simulink model "libdumbac"  (R2020a)
settings: Solver=FixedStepDiscrete  StartTime=0.0  StopTime=86400  FixedStep=10  RelTol=1e-3
values from neighbouring files (symbols this model uses):
  conE = [ ... (first row only)    [acMdl.m]
  t0filt = Hd.Numerator ./ sum(Hd.Numerator)    [acMdl.m]
libraries: mpclib x1, cstblocks x1
settings Model: Creator=iorioikawa  LastModifiedBy=iorioikawa
settings DataIOCC: SaveOutput=off  SaveTime=off
settings OptimizationCC: DefaultParameterBehavior=Inlined  UseDivisionForNetSlopeComputation=on  GainParamInheritBuiltInType=on  UseFloatMulNetSlope=on  InlineInvariantSignals=on  PassReuseOutputArgsAs=Individual arguments  ZeroExternalMemoryAtStartup=off  ZeroInternalMemoryAtStartup=off  NoFixptDivByZeroProtection=on  EfficientFloat2IntCast=on  LifeSpan=365  OptimizeBlockOrder=speed  DifferentSizesBufferReuse=on  EfficientTunableParamExpr=on
settings DebuggingCC: ParameterTunabilityLossMsg=error
settings HardwareCC: ProdBitPerPointer=32  ProdBitPerSizeT=32  ProdBitPerPtrDiffT=32  ProdLargestAtomicInteger=Long  ProdWordSize=32  ProdLongLongMode=on  ProdHWDeviceType=ARM Compatible->ARM 7
settings SFSimCC: MATLABDynamicMemAlloc=off
settings RTWCC: SystemTargetFile=ert.tlc  GenCodeOnly=on  TemplateMakefile=ert_default_tmf  TargetLang=C++
settings CodeAppCC: ForceParamTrailComments=on  IgnoreCustomStorageClasses=off  OperatorAnnotations=on  SimulinkDataObjDesc=on  SFDataObjDesc=on  CustomSymbolStrGlobalVar=rt$N$M  CustomSymbolStrType=$N$M  CustomSymbolStrFcn=$N$M$F  CustomSymbolStrMacro=$N$M  InsertBlockDesc=on
settings ERTTargetCC: TargetLangStandard=C++03 (ISO)  GenerateSampleERTMain=on  IncludeMdlTerminateFcn=off  CombineSignalStateStructs=on  SupportAbsoluteTime=off  MultiInstanceERTCode=on  CodeInterfacePackaging=C++ class  SupportComplex=off  SupportNonInlinedSFcns=on  InlinedParameterPlacement=NonHierarchical  RootIOFormat=Structure reference  RTWCAPISignals=on  ERTCustomFileTemplate=example_file_process.tlc  ERTFilePackagingFormat=CompactWithDataFile  IndentStyle=Allman  IndentSize=4

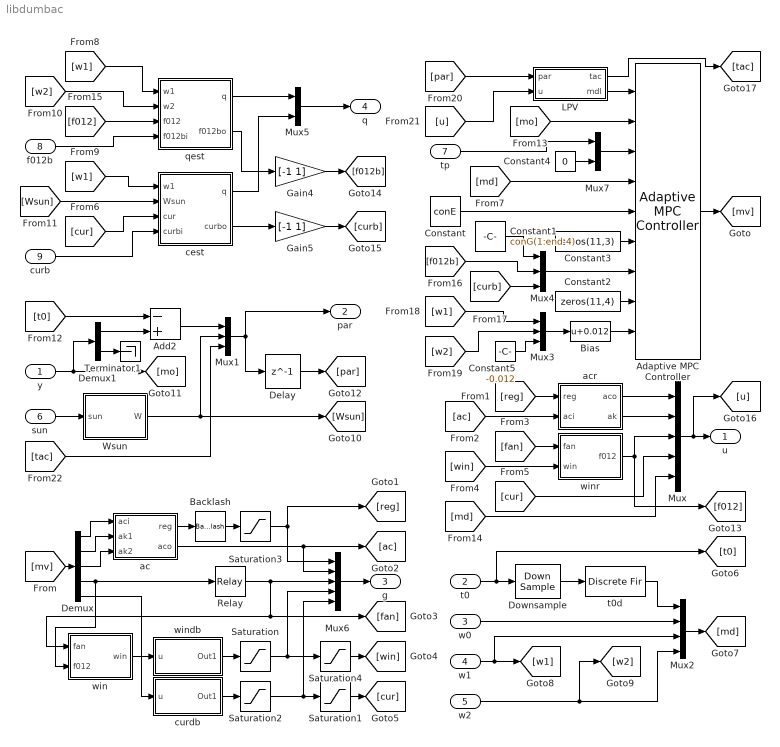
== system libdumbac ==
  y : Inport  OutDataTypeStr=double  PortDimensions=2  SampleTime=10
  t0 : Inport  Port=2  OutDataTypeStr=double  PortDimensions=1  SampleTime=10
  w0 : Inport  Port=3  OutDataTypeStr=double  PortDimensions=1  SampleTime=10
  w1 : Inport  Port=4  OutDataTypeStr=double  PortDimensions=1  SampleTime=10
  w2 : Inport  Port=5  OutDataTypeStr=double  PortDimensions=1  SampleTime=10
  sun : Inport  Port=6  OutDataTypeStr=double  PortDimensions=3  SampleTime=10
  tp : Inport  Port=7  OutDataTypeStr=double  PortDimensions=2  SampleTime=10
  f012b : Inport  Port=8  OutDataTypeStr=double  PortDimensions=2  SampleTime=10
  curb : Inport  Port=9  OutDataTypeStr=double  PortDimensions=2  SampleTime=10
  Adaptive MPC Controller : mpclib/Adaptive MPC Controller  SCDEnableBlockLinearizationSpecification=on  mpcobj=Gdsam  enable_value=0  updateMPCinCallerWorkspace=on  md_inport=on  mv_inport=off  uref_inport=off  return_cost=off  return_mvseq=off  return_qpstatus=off  return_xseq=off  return_state=off  return_ovseq=off  state_inport=off  isltv_plant=off  umin_inport=off  umax_inport=off  ymin_inport=off  ymax_inport=off  cc_inport=on  ywt_inport=on  uwt_inport=off  duwt_inport=off  rhoeps_inport=off  pm_inport=off  MaximumP=10  HorizonChoice=FixedHorizon  BlockDataType=double  SampleTimeInherited=off  switch_inport=off
  Add2 : Sum  Inputs=-+
  Backlash : Backlash  BacklashWidth=0.005
  Bias : Bias  Bias=0.012
  Constant : Constant  Value=conE
  Constant1 : Constant  Value=conG(1:end-4)
  Constant2 : Constant  Value=zeros(11,4)
  Constant3 : Constant  Value=zeros(11,3)
  Constant4 : Constant  Value=0
  Constant5 : Constant  Value=-0.012
  Delay : Delay  DelayLength=1  InitialCondition=0
  Demux : Demux  Outputs=5
  Demux1 : Demux  Outputs=2
  Downsample : DownSample  N=60
  Gain4 : Gain  Gain=[-1 1]
  Gain5 : Gain  Gain=[-1 1]
  LPV : Subsystem
  Mux : Mux  Inputs=5
  Mux1 : Mux  Inputs=3
  Mux2 : Mux
  Mux3 : Mux  Inputs=3
  Mux4 : Mux  Inputs=3
  Mux5 : Mux  Inputs=2
  Mux6 : Mux  Inputs=5
  Mux7 : Mux  Inputs=2
  Relay : Relay  OnSwitchValue=0.2  OffSwitchValue=0.1
  Saturation : Saturate  UpperLimit=1  LowerLimit=-0.1
  Saturation1 : Saturate  UpperLimit=1  LowerLimit=0
  Saturation2 : Saturate  UpperLimit=1  LowerLimit=-0.1
  Saturation3 : Saturate  UpperLimit=2  LowerLimit=0
  Saturation4 : Saturate  UpperLimit=1  LowerLimit=0
  Terminator1 : Terminator
  Wsun : MATLAB Function  TreatAsAtomicUnit=on
  ac : Subsystem
  acr : MATLAB Function  TreatAsAtomicUnit=on
  cest : Subsystem
  curdb : Subsystem
  qest : Subsystem
  t0d : DiscreteFir  Coefficients=t0filt
  win : MATLAB Function  TreatAsAtomicUnit=on
  windb : Subsystem
  winr : MATLAB Function  TreatAsAtomicUnit=on
  u : Outport  OutDataTypeStr=double  PortDimensions=9  SampleTime=10
  par : Outport  Port=2  OutDataTypeStr=double  PortDimensions=3  SampleTime=10
  g : Outport  Port=3  OutDataTypeStr=double  PortDimensions=8  SampleTime=10
  q : Outport  Port=4  OutDataTypeStr=double  PortDimensions=2  SampleTime=10
  wires:
  Mux1/1 -> par/1, Delay/1
  w1/1 -> [w1], Mux2/3
  w2/1 -> Mux2/4, [w2]
  Mux3/1 -> Bias/1
  Add2/1 -> Mux1/1
  t0d/1 -> Mux2/1
  Bias/1 -> Adaptive MPC Controller/9
  y/1 -> Demux1/1, [mo]
  w0/1 -> Mux2/2
  t0/1 -> [t0], Downsample/1
  Demux1/1 -> Add2/2
  sun/1 -> Wsun/1(sun)
  Demux1/2 -> Terminator1/1
  Mux/1 -> [u], u/1
  Delay/1 -> [par]
  acr/1(aco) -> Mux/1
  acr/2(ak) -> Mux/2
  Demux/5 -> curdb/1(u)
  Demux/4 -> win/2(f012), Relay/1
  Relay/1 -> Mux6/3, [fan], win/1(fan)
  win/1(win) -> windb/1(u)
  curdb/1(Out1) -> Saturation2/1
  windb/1(Out1) -> Saturation/1
  Saturation/1 -> Saturation4/1, Mux6/4
  ac/2(aco) -> [ac], Mux6/2
  Saturation2/1 -> Mux6/5, Saturation1/1
  Backlash/1 -> Saturation3/1
  winr/1(f012) -> Mux/3, [f012]
  Mux6/1 -> g/1
  Saturation3/1 -> [reg], Mux6/1
  Demux/1 -> ac/1(aci)
  Demux/2 -> ac/2(ak1)
  ac/1(reg) -> Backlash/1
  Saturation1/1 -> [cur]
  Downsample/1 -> t0d/1
  f012b/1 -> qest/4(f012bi)
  Constant/1 -> Adaptive MPC Controller/5
  Constant2/1 -> Adaptive MPC Controller/8
  Constant3/1 -> Adaptive MPC Controller/6
  Mux4/1 -> Adaptive MPC Controller/7
  Constant1/1 -> Mux4/1
  qest/2(f012bo) -> Gain4/1
  cest/2(curbo) -> Gain5/1
  Mux5/1 -> q/1
  qest/1(q) -> Mux5/1
  cest/1(q) -> Mux5/2
  curb/1 -> cest/4(curbi)
  Adaptive MPC Controller/1 -> [mv]
  [mv] -> Demux/1
  [reg] -> acr/1(reg)
  [ac] -> acr/2(aci)
  [fan] -> winr/1(fan)
  Saturation4/1 -> [win]
  [win] -> winr/2(win)
  [cur] -> cest/3(cur)
  [cur] -> Mux/4
  Mux2/1 -> [md]
  [md] -> Adaptive MPC Controller/4
  [w1] -> qest/1(w1)
  [w1] -> cest/1(w1)
  [w2] -> qest/2(w2)
  Wsun/1(W) -> [Wsun], Mux1/2
  [Wsun] -> cest/2(Wsun)
  [t0] -> Add2/1
  [mo] -> Adaptive MPC Controller/2
  [md] -> Mux/5
  [f012] -> qest/3(f012)
  Gain4/1 -> [f012b]
  [f012b] -> Mux4/2
  Gain5/1 -> [curb]
  [curb] -> Mux4/3
  [w1] -> Mux3/1
  [w2] -> Mux3/2
  [par] -> LPV/1(par)
  LPV/2(mdl) -> Adaptive MPC Controller/1
  Demux/3 -> ac/3(ak2)
  [u] -> LPV/2(u)
  LPV/1(tac) -> [tac]
  [tac] -> Mux1/3
  Mux7/1 -> Adaptive MPC Controller/3
  tp/1 -> Mux7/1
  Constant4/1 -> Mux7/2
  Constant5/1 -> Mux3/3

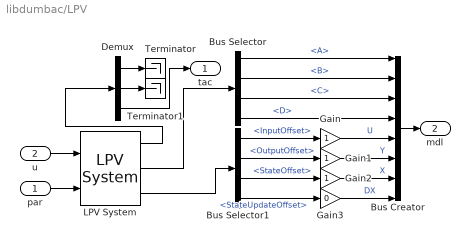
== system libdumbac/LPV ==
  par : Inport
  u : Inport  Port=2
  Bus Creator : BusCreator  Inputs=8
  Bus Selector : BusSelector  OutputSignals=A,B,C,D
  Bus Selector1 : BusSelector  OutputSignals=InputOffset,OutputOffset,StateOffset,StateUpdateOffset
  Demux : Demux  Outputs=3
  Gain : Gain
  Gain1 : Gain
  Gain2 : Gain
  Gain3 : Gain  Gain=0
  LPV System : cstblocks/Linear Parameter Varying/LPV System  sys=Gds  x0=0  uOffset=0  yOffset=0  xOffset=0  opEquilOption=on  dxOffset=0  sysFixedOption=Use the first model in state-space array  sysFixed=[]  AFixed=true  BFixed=false  CFixed=true  DFixed=true  uDelayFixed=true  yDelayFixed=true  iDelayFixed=true  IMethod=Linear  EMethod=Clip  IndexSearch=Linear search  IndexBegin=on  OutputX=off  OutputXdot=off  OutputLTI=on  OutputOP=on  DataType=double  SimMode=Interpreted execution  InitBufferSize=1024  FixedBuffer=off
      settings: SourceProductBaseCode=CT
  Terminator : Terminator
  Terminator1 : Terminator
  tac : Outport
  mdl : Outport  Port=2
  wires:
  u/1 -> LPV System/1
  LPV System/1 -> Demux/1
  Bus Selector/1 -> Bus Creator/1  "<A>"
  Bus Selector1/3 -> Gain2/1  "<StateOffset>"
  Bus Selector/2 -> Bus Creator/2  "<B>"
  Gain2/1 -> Bus Creator/7  "X"
  LPV System/3 -> Bus Selector1/1
  Gain1/1 -> Bus Creator/6  "Y"
  Bus Selector1/1 -> Gain/1  "<InputOffset>"
  Bus Selector/4 -> Bus Creator/4  "<D>"
  par/1 -> LPV System/2
  Gain/1 -> Bus Creator/5  "U"
  LPV System/2 -> Bus Selector/1
  Gain3/1 -> Bus Creator/8  "DX"
  Bus Selector1/2 -> Gain1/1  "<OutputOffset>"
  Bus Selector/3 -> Bus Creator/3  "<C>"
  Bus Creator/1 -> mdl/1
  Bus Selector1/4 -> Gain3/1  "<StateUpdateOffset>"
  Demux/1 -> Terminator/1
  Demux/2 -> Terminator1/1
  Demux/3 -> tac/1

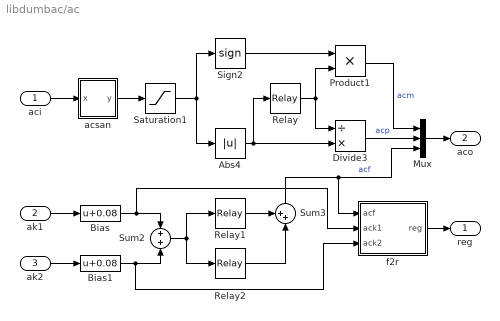
== system libdumbac/ac ==
  aci : Inport
  ak1 : Inport  Port=2
  ak2 : Inport  Port=3
  Abs4 : Abs
  Bias : Bias  Bias=0.08
  Bias1 : Bias  Bias=0.08
  Divide3 : Product  Inputs=/*
  Mux : Mux  Inputs=3
  Product1 : Product
  Relay : Relay  OnSwitchValue=1  OffSwitchValue=0.9  OnOutputValue=2  OffOutputValue=1
  Relay1 : Relay  OnSwitchValue=0.8  OffSwitchValue=0.7
  Relay2 : Relay  OnSwitchValue=0.65  OffSwitchValue=0.55
  Saturation1 : Saturate  UpperLimit=2  LowerLimit=-2
  Sign2 : Signum
  Sum2 : Sum  Inputs=+|+
  Sum3 : Sum  Inputs=++|
  acsan : Subsystem
  f2r : MATLAB Function  TreatAsAtomicUnit=on
  reg : Outport
  aco : Outport  Port=2
  wires:
  f2r/1(reg) -> reg/1
  acsan/1(y) -> Saturation1/1
  aci/1 -> acsan/1(x)
  Saturation1/1 -> Abs4/1, Sign2/1
  Abs4/1 -> Relay/1, Divide3/2
  Divide3/1 -> Mux/2  "acp"
  Product1/1 -> Mux/1  "acm"
  Mux/1 -> aco/1
  Relay/1 -> Divide3/1, Product1/2
  Sign2/1 -> Product1/1
  ak1/1 -> Bias/1
  ak2/1 -> Bias1/1
  Sum2/1 -> Relay1/1, Relay2/1
  Relay1/1 -> Sum3/1
  Relay2/1 -> Sum3/2
  Sum3/1 -> f2r/1(acf), Mux/3  "acf"
  Bias/1 -> f2r/2(ack1), Sum2/1
  Bias1/1 -> f2r/3(ack2), Sum2/2

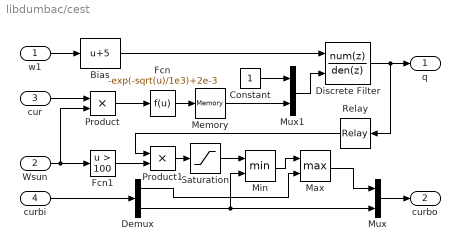
== system libdumbac/cest ==
  w1 : Inport
  Wsun : Inport  Port=2
  cur : Inport  Port=3
  curbi : Inport  Port=4
  Bias : Bias  Bias=5
  Constant : Constant
  Demux : Demux  Outputs=2
  Discrete Filter : DiscreteFilter  Numerator=9e-4  DenominatorSource=Input port  Denominator=[1 -1]  a0EqualsOne=on
      settings: InputPortMap=u0,p3
  Fcn : Fcn  Expr=-exp(-sqrt(u)/1e3)+2e-3
  Fcn1 : Fcn  Expr=u > 100
  Max : MinMax  Function=max  Inputs=2
  Memory : Memory
  Min : MinMax  Inputs=2
  Mux : Mux  Inputs=2
  Mux1 : Mux  Inputs=2
  Product : Product
  Product1 : Product
  Relay : Relay  OnSwitchValue=2  OffSwitchValue=0.2  OnOutputValue=0.15
  Saturation : Saturate  UpperLimit=1  LowerLimit=0
  q : Outport
  curbo : Outport  Port=2
  wires:
  Discrete Filter/1 -> q/1, Relay/1
  w1/1 -> Bias/1
  curbi/1 -> Demux/1
  Mux/1 -> curbo/1
  Demux/2 -> Mux/2, Min/2
  Demux/1 -> Max/2
  Max/1 -> Mux/1
  Min/1 -> Max/1
  Fcn/1 -> Memory/1
  Mux1/1 -> Discrete Filter/2
  Constant/1 -> Mux1/1
  Memory/1 -> Mux1/2
  Bias/1 -> Discrete Filter/1
  Product/1 -> Fcn/1
  Wsun/1 -> Product/2, Fcn1/1
  Relay/1 -> Product1/1
  Fcn1/1 -> Product1/2
  cur/1 -> Product/1
  Product1/1 -> Saturation/1
  Saturation/1 -> Min/1

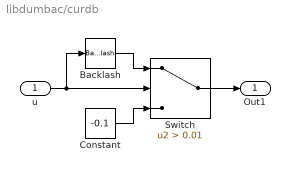
== system libdumbac/curdb ==
  u : Inport
  Backlash : Backlash  BacklashWidth=0.05
  Constant : Constant  Value=-0.1
  Switch : Switch  Criteria=u2 > Threshold  Threshold=0.01
  Out1 : Outport
  wires:
  Constant/1 -> Switch/3
  Switch/1 -> Out1/1
  Backlash/1 -> Switch/1
  u/1 -> Backlash/1, Switch/2

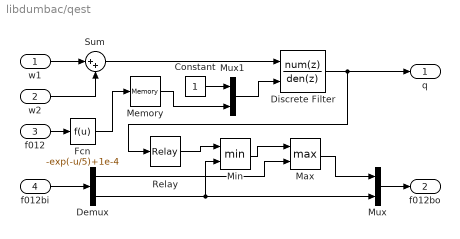
== system libdumbac/qest ==
  w1 : Inport
  w2 : Inport  Port=2
  f012 : Inport  Port=3
  f012bi : Inport  Port=4
  Constant : Constant
  Demux : Demux  Outputs=2
  Discrete Filter : DiscreteFilter  Numerator=1e-3  DenominatorSource=Input port  Denominator=[1 -1]  a0EqualsOne=on
      settings: InputPortMap=u0,p3
  Fcn : Fcn  Expr=-exp(-u/5)+1e-4
  Max : MinMax  Function=max  Inputs=2
  Memory : Memory
  Min : MinMax  Inputs=2
  Mux : Mux  Inputs=2
  Mux1 : Mux  Inputs=2
  Relay : Relay  OnSwitchValue=2  OffSwitchValue=0.2
  Sum : Sum  Inputs=|++
  q : Outport
  f012bo : Outport  Port=2
  wires:
  Discrete Filter/1 -> q/1, Relay/1
  w1/1 -> Sum/1
  w2/1 -> Sum/2
  f012/1 -> Fcn/1
  Relay/1 -> Min/1
  f012bi/1 -> Demux/1
  Mux/1 -> f012bo/1
  Demux/2 -> Mux/2, Min/2
  Demux/1 -> Max/2
  Max/1 -> Mux/1
  Min/1 -> Max/1
  Fcn/1 -> Memory/1
  Mux1/1 -> Discrete Filter/2
  Constant/1 -> Mux1/1
  Memory/1 -> Mux1/2
  Sum/1 -> Discrete Filter/1

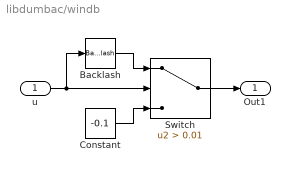
== system libdumbac/windb ==
  u : Inport
  Backlash : Backlash  BacklashWidth=0.05
  Constant : Constant  Value=-0.1
  Switch : Switch  Criteria=u2 > Threshold  Threshold=0.01
  Out1 : Outport
  wires:
  Constant/1 -> Switch/3
  Switch/1 -> Out1/1
  Backlash/1 -> Switch/1
  u/1 -> Backlash/1, Switch/2

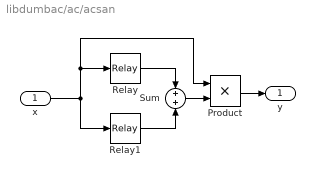
== system libdumbac/ac/acsan ==
  x : Inport
  Product : Product
  Relay : Relay  OnSwitchValue=0.4  OffSwitchValue=0.2
  Relay1 : Relay  OnSwitchValue=-0.2  OffSwitchValue=-0.4  OnOutputValue=0  OffOutputValue=1
  Sum : Sum  Inputs=+|+
  y : Outport
  wires:
  Product/1 -> y/1
  Sum/1 -> Product/2
  Relay1/1 -> Sum/2
  Relay/1 -> Sum/1
  x/1 -> Relay1/1, Product/1, Relay/1

== matlab function libdumbac/acr ==
  data: reg input; aci input; aco output; ak output
function [aco, ak] = acr(reg, aci)

aco = aci(1)*aci(2);
if aci(3) == 0
    ak1 = 0.4;
    ak2 = 0.1;
elseif aci(3) == 1
    ak1 = reg(1)*0.5+0.4;
    ak2 = reg(2)*0.5+0.1;
    if ak1 > ak2
        ak1 = 1 - ak2;
    else
        ak2 = 1 - ak1;
    end
else
    ak1 = reg(1)*0.25+0.4;
    ak2 = reg(2)*0.25+0.1;
    if ak1 > ak2
        ak1 = 1 - ak2;
    else
        ak2 = 1 - ak1;
    end
end
ak = [ak1, ak2] - 0.08;

end

== matlab function libdumbac/win ==
  data: fan input; win output; f012 input
function win  = win(fan, f012)

if fan == 0
    win = f012 ./ 0.2;
else
    win = f012;
end

end

== matlab function libdumbac/Wsun ==
  data: sun input; W output
function W = Wsun(sun)

ton = sun(1);
toff = sun(2);
ta = ton - (toff+ton).*0.1;
tb = toff - (toff+ton).*0.1;
sr = 1.4;
uvi = sun(3);
W = 140.*uvi./(1+exp(-sr.*ta))./(1+exp(-sr.*tb));

== matlab function libdumbac/ac/f2r ==
  data: reg output; acf input; ack1 input; ack2 input
function reg = f2r(acf, ack1, ack2)

if acf == 0
    reg = [0 0];
else
    reg = [(ack1-0.4)*3 (ack2-0.1)*6];
    if reg(1) > 1
        reg(1) = 1;
    end
    if reg(2) > 1
        reg(2) = 1;
    end
end

end

== matlab function libdumbac/winr ==
  data: fan input; f012 output; win input
function f012  = winr(fan, win)

if fan == 0
    f012 = 0.2 .* win;
else
    f012 = win;
end

end
